simulink library "INT_CoVMD_TrqLeadCoord"  (R2016b)
settings: Solver=VariableStepAuto  StartTime=0.0  StopTime=10.0  RelTol=1e-3
settings Model: Creator=liutao  LastModifiedBy=liutao

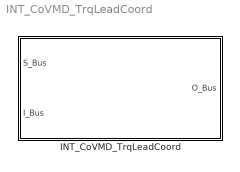
== system INT_CoVMD_TrqLeadCoord ==
  INT_CoVMD_TrqLeadCoord : Subsystem

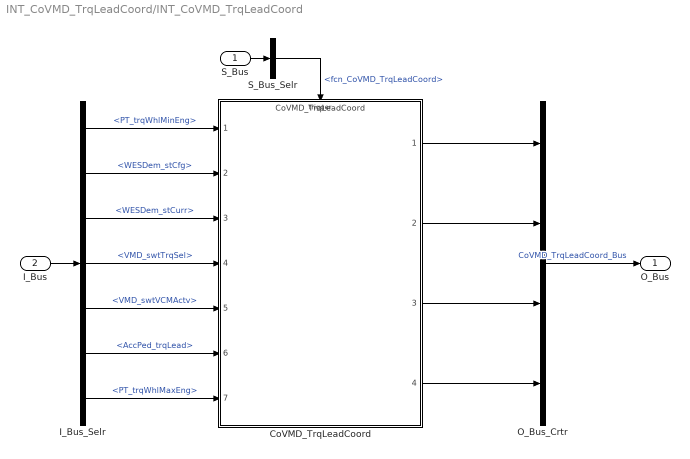
== system INT_CoVMD_TrqLeadCoord/INT_CoVMD_TrqLeadCoord ==
  S_Bus : Inport
  I_Bus : Inport  Port=2
  CoVMD_TrqLeadCoord : ModelReference  ModelNameDialog=CoVMD_TrqLeadCoord  SimulationMode=Normal  ModelReferenceVersion=1.14  TriggerPortName=function  TriggerPortTriggerType=function-call  TriggerPortStatesWhenEnabling=held
  I_Bus_Selr : BusSelector  OutputSignals=PT_trqWhlMinEng,WESDem_stCfg,WESDem_stCurr,VMD_swtTrqSel,VMD_swtVCMActv,AccPed_trqLead,PT_trqWhlMaxEng
  O_Bus_Crtr : BusCreator  Inputs=4
  S_Bus_Selr : BusSelector  OutputSignals=fcn_CoVMD_TrqLeadCoord
  O_Bus : Outport
  wires:
  S_Bus_Selr/1 -> CoVMD_TrqLeadCoord/Trigger  "<fcn_CoVMD_TrqLeadCoord>"
  S_Bus/1 -> S_Bus_Selr/1
  I_Bus/1 -> I_Bus_Selr/1
  I_Bus_Selr/1 -> CoVMD_TrqLeadCoord/1  "<PT_trqWhlMinEng>"
  I_Bus_Selr/2 -> CoVMD_TrqLeadCoord/2  "<WESDem_stCfg>"
  I_Bus_Selr/3 -> CoVMD_TrqLeadCoord/3  "<WESDem_stCurr>"
  I_Bus_Selr/4 -> CoVMD_TrqLeadCoord/4  "<VMD_swtTrqSel>"
  I_Bus_Selr/5 -> CoVMD_TrqLeadCoord/5  "<VMD_swtVCMActv>"
  I_Bus_Selr/6 -> CoVMD_TrqLeadCoord/6  "<AccPed_trqLead>"
  I_Bus_Selr/7 -> CoVMD_TrqLeadCoord/7  "<PT_trqWhlMaxEng>"
  O_Bus_Crtr/1 -> O_Bus/1  "CoVMD_TrqLeadCoord_Bus"
  CoVMD_TrqLeadCoord/1 -> O_Bus_Crtr/1
  CoVMD_TrqLeadCoord/2 -> O_Bus_Crtr/2
  CoVMD_TrqLeadCoord/3 -> O_Bus_Crtr/3
  CoVMD_TrqLeadCoord/4 -> O_Bus_Crtr/4
